simulink model "EV_thermal_charger_2015a_20200311"  (R2015a)
settings: Solver=ode3  StartTime=0.0  StopTime=1800  FixedStep=sampling_time  RelTol=1e-3
PreLoadFcn:
  | run('init_setting.m')
PostLoadFcn:
  | set_param(gcs, 'SimulationCommand', 'update');
  | load('save_param/save_P_Charger', 'P_Charger');
  | load('save_param/save_T_User_set_temp_degC','T_User_set_temp_degC');
  | load('save_param/save_ENV_PNT_PTTH_Temp_add_degC','ENV_PNT_PTTH_Temp_add_degC');
  | load('save_param/save_ENV_PNT_CABIN_Temp_add_degC','ENV_PNT_CABIN_Temp_add_degC');
  | load('save_param/save_ENV_PNT_PHI_Sunlight_W','ENV_PNT_PHI_Sunlight_W');
  | load('save_param/save_ENV_PNT_Outside_Temp_ini_degC','ENV_PNT_Outside_Temp_ini_degC');
undefined symbols (not defined in the file or in its folder): BK_PNT_Pow_UL, BK_PNT_ReGene_vel_limit_DN_kmph, BK_PNT_ReGene_vel_limit_UP_kmph, BK_PNT_Tau_brake, Brk_LL, Brk_PGain, Brk_UL, BT_PNT_Hi_C_pol_hi_batt, BT_PNT_Hi_Capa_hi_batt_F, BT_PNT_Hi_ocv_SOC_hi_batt_OCV_V_table, BT_PNT_Hi_ocv_SOC_hi_batt_OCV_V_table_x_SOC, BT_PNT_Hi_R_hi_batt_cell, BT_PNT_Hi_R_pol_hi_batt, BT_PNT_Hi_SOC_MAX_hi_batt, BT_PNT_Hi_SOC_MIN_hi_batt, BT_PNT_Hi_SOC_START_hi_batt, BT_PNT_Lo_Capa_lo_batt_F, BT_PNT_Lo_ocv_SOC_lo_batt_OCV_V_table, BT_PNT_Lo_ocv_SOC_lo_batt_OCV_V_table_x_SOC, BT_PNT_Lo_R_lo_batt_ohm, BT_PNT_Lo_SOC_MAX_lo_batt, BT_PNT_Lo_SOC_MIN_lo_batt, BT_PNT_Lo_SOC_START_lo_batt, BTTH_CNT_P_BT_Heater_W, BTTH_CNT_P_BT_Heater_W_x_BTCells_degC, BTTH_CNT_Voltage_BTFan_V, BTTH_CNT_Voltage_BTFan_V_x_BTCells_degC, BTTH_PNT_BT_Heat_Resi_KpW, BTTH_PNT_BT_Heat_Resi_KpW_x_Wind_m3ps, BTTH_PNT_BT_Heater2BTCells_Heat_Resi_KpW, BTTH_PNT_BT_Heater_Heat_Capa_JpK, BTTH_PNT_BTBlock2BTAir_Heat_Resi_KpW, BTTH_PNT_BTBlock_Heat_Capa_JpK, BTTH_PNT_BTCells2BTBlock_Heat_Resi_KpW, BTTH_PNT_BTCells_Heat_Capa_JpK, BTTH_PNT_v_BTFan_Wind_vel_mps, BTTH_PNT_v_BTFan_Wind_vel_mps_x_V_BTFan, CATH_CNT_P_Aircon_W_LL, CATH_CNT_P_Aircon_W_UL, CATH_CNT_P_Gain_Aircon, CATH_CNT_P_Gain_PTC_Heater, CATH_CNT_P_Gain_SeatHT, CATH_CNT_P_PTC_Heater, CATH_CNT_P_PTC_Heater_W_LL, CATH_CNT_P_PTC_Heater_W_UL, CATH_CNT_P_PTC_Heater_x_T_Outside_temp_degC, CATH_CNT_P_SeatHT_W_LL, CATH_CNT_P_SeatHT_W_UL, CATH_CNT_PGain_Temp_blowout, CATH_CNT_T_Aircon_Indoor_degC, CATH_CNT_T_Aircon_Indoor_degC_x_T_blowout_degC, CATH_CNT_T_PTC_Heater_degC_UL, CATH_CNT_T_SeatHT_Temp_degC, CATH_CNT_T_SeatHT_Temp_degC_x_T_blowout_degC, CATH_CNT_V_HVAC_Fan, CATH_CNT_V_HVAC_Fan_x_T_blowout_degC, CATH_CNT_V_RDFan_V, CATH_CNT_V_RDFan_x_P_Aircon_W, CATH_PNT_Air_Convection_Heat_Resi_KpW, CATH_PNT_Air_Convection_Heat_Resi_x_mps ... (+141)
undefined symbols (not defined in the file): ACC_D_Gain, ACC_I_Gain, ACC_P_Gain
libraries: METI_Lib_vehicle_model x52, simulink x35
(part 6 of 6)

== system EV_thermal_charger_2015a_20200311/Vehicle/CATH_PNT/CABIN/WALL/CABIN_Wall_Heat_Resistance/Heat_Resistance_Calc/R3 ==
  S_Heat_Conduction_m2 : Inport
  wall_heat_resi : Inport  Port=2
  Divide : Product  Inputs=*/
  R3 : Outport
  wires:
  S_Heat_Conduction_m2/1 -> Divide/2
  wall_heat_resi/1 -> Divide/1
  Divide/1 -> R3/1

== system EV_thermal_charger_2015a_20200311/Vehicle/CATH_PNT/CABIN/WALL/CABIN_Wall_Heat_Resistance/Heat_Resistance_Calc/Subsystem ==
  note: 直列抵抗部分の
      | 抵抗値計算
      | 単純和
  note: 並列抵抗部分の
      | 抵抗値計算
  R2 : Inport
  R1 : Inport  Port=2
  R3 : Inport  Port=3
  Add : Sum
  Add1 : Sum
  Divide : Product  Inputs=*/
  Product : Product
  R_total : Outport
  wires:
  R1/1 -> Add/1, Product/1
  R2/1 -> Product/2, Add/2
  Product/1 -> Divide/1
  Add/1 -> Divide/2
  Divide/1 -> Add1/1
  Add1/1 -> R_total/1
  R3/1 -> Add1/2

== system EV_thermal_charger_2015a_20200311/Vehicle/CATH_PNT/CABIN/WALL/CABIN_Wall_Heat_Resistance/Heat_Resistance_Calc/Subsystem1 ==
  T_In1_K : Inport
  T_Glass_center_K : Inport  Port=2
  R3 : Inport  Port=3
  R_total : Inport  Port=4
  Add : Sum
  Divide : Product  Inputs=*/
  Product : Product
  Subtract : Sum  Inputs=-+
  T_Glass_surface_K : Outport
  wires:
  T_Glass_center_K/1 -> Subtract/2
  T_In1_K/1 -> Add/1, Subtract/1
  R3/1 -> Divide/1
  R_total/1 -> Divide/2
  Subtract/1 -> Product/1
  Divide/1 -> Product/2
  Product/1 -> Add/2
  Add/1 -> T_Glass_surface_K/1

== system EV_thermal_charger_2015a_20200311/Vehicle/CATH_PNT/CABIN/WALL/CABIN_Wall_Heat_Resistance/Heat_Resistance_Calc/Subsystem2 ==

== system EV_thermal_charger_2015a_20200311/Vehicle/CATH_PNT/CABIN/WALL/CABIN_Wall_Heat_Resistance1/Heat_Resistance_Calc/R1 ==
  note: [K/W]
  note: [W/m2K]
  emissivity : Inport
  T_In1_K : Inport  Port=2
  T_Glass_surface_K : Inport  Port=3
  S_Heat_Conduction_m2 : Inport  Port=4
  Add : Sum
  Add1 : Sum
  Constant : Constant  Value=sigma_Stefan_Boltzmann
  Divide : Product  Inputs=/*
  Math Function : Math  Operator=magnitude^2  SaturateOnIntegerOverflow=on
  Math Function1 : Math  Operator=magnitude^2  SaturateOnIntegerOverflow=on
  Product : Product  Inputs=3
  Product1 : Product
  R1 : Outport
  wires:
  T_Glass_surface_K/1 -> Add1/2, Math Function1/1
  Math Function/1 -> Add/1
  Math Function1/1 -> Add/2
  T_In1_K/1 -> Add1/1, Math Function/1
  Add/1 -> Product/2
  Add1/1 -> Product/3
  Product1/1 -> Product/1
  Product/1 -> Divide/1
  Divide/1 -> R1/1
  S_Heat_Conduction_m2/1 -> Divide/2
  Constant/1 -> Product1/1
  emissivity/1 -> Product1/2

== system EV_thermal_charger_2015a_20200311/Vehicle/CATH_PNT/CABIN/WALL/CABIN_Wall_Heat_Resistance1/Heat_Resistance_Calc/R2 ==
  note: [K/W]
  note: [m2K/W]
  note: ユルゲスの実験式による
      | 対流の熱伝達率[W/m2K]を逆数にして
      | 熱抵抗[m2K/W]にしたもの
  V_wind_mps : Inport
  S_Heat_Conduction_m2 : Inport  Port=2
  Abs : Abs
  Air_Convection_Heat_Resi : Lookup_n-D  NumberOfTableDimensions=1  BreakpointsForDimension1=CATH_PNT_Air_Convection_Heat_Resi_x_mps  Table=CATH_PNT_Air_Convection_Heat_Resi_KpW  InternalRulePriority=Speed  RndMeth=Simplest  InputSameDT=on
  Divide : Product  Inputs=*/
  R2 : Outport
  wires:
  V_wind_mps/1 -> Abs/1
  Air_Convection_Heat_Resi/1 -> Divide/1
  Abs/1 -> Air_Convection_Heat_Resi/1
  S_Heat_Conduction_m2/1 -> Divide/2
  Divide/1 -> R2/1

== system EV_thermal_charger_2015a_20200311/Vehicle/CATH_PNT/CABIN/WALL/CABIN_Wall_Heat_Resistance1/Heat_Resistance_Calc/R3 ==
  S_Heat_Conduction_m2 : Inport
  wall_heat_resi : Inport  Port=2
  Divide : Product  Inputs=*/
  R3 : Outport
  wires:
  S_Heat_Conduction_m2/1 -> Divide/2
  wall_heat_resi/1 -> Divide/1
  Divide/1 -> R3/1

== system EV_thermal_charger_2015a_20200311/Vehicle/CATH_PNT/CABIN/WALL/CABIN_Wall_Heat_Resistance1/Heat_Resistance_Calc/Subsystem ==
  note: 直列抵抗部分の
      | 抵抗値計算
      | 単純和
  note: 並列抵抗部分の
      | 抵抗値計算
  R2 : Inport
  R1 : Inport  Port=2
  R3 : Inport  Port=3
  Add : Sum
  Add1 : Sum
  Divide : Product  Inputs=*/
  Product : Product
  R_total : Outport
  wires:
  R1/1 -> Add/1, Product/1
  R2/1 -> Product/2, Add/2
  Product/1 -> Divide/1
  Add/1 -> Divide/2
  Divide/1 -> Add1/1
  Add1/1 -> R_total/1
  R3/1 -> Add1/2

== system EV_thermal_charger_2015a_20200311/Vehicle/CATH_PNT/CABIN/WALL/CABIN_Wall_Heat_Resistance1/Heat_Resistance_Calc/Subsystem1 ==
  T_In1_K : Inport
  T_Glass_center_K : Inport  Port=2
  R3 : Inport  Port=3
  R_total : Inport  Port=4
  Add : Sum
  Divide : Product  Inputs=*/
  Product : Product
  Subtract : Sum  Inputs=-+
  T_Glass_surface_K : Outport
  wires:
  T_Glass_center_K/1 -> Subtract/2
  T_In1_K/1 -> Add/1, Subtract/1
  R3/1 -> Divide/1
  R_total/1 -> Divide/2
  Subtract/1 -> Product/1
  Divide/1 -> Product/2
  Product/1 -> Add/2
  Add/1 -> T_Glass_surface_K/1

== system EV_thermal_charger_2015a_20200311/Vehicle/CATH_PNT/CABIN/WALL/CABIN_Wall_Heat_Resistance1/Heat_Resistance_Calc/Subsystem2 ==
